simulink model "bustestsysa"  (Simulink 9.3)
settings: Solver=ode15s  StartTime=0.0  StopTime=0.08  RelTol=1e-3  AbsTol=1e-6
libraries: powerlib x113
settings Model: Creator=Dr. Lotfifard  LastModifiedBy=renji  ExtModeTrigMode=oneshot  ExtModeArmWhenConnect=off
settings SolverCC: AutoScaleAbsTol=off
settings OptimizationCC: BlockReduction=off  BooleanDataType=off  ExpressionDepthLimit=2147483647
settings DebuggingCC: SaveWithParameterizedLinksMsg=none  SignalResolutionControl=TryResolveAllWithWarning  MultiTaskDSMMsg=warning  MultiTaskCondExecSysMsg=none  StateNameClashWarn=warning
settings HardwareCC: TargetUnknown=on
settings GRTTargetCC: GeneratePreprocessorConditionals=Disable all
settings SimscapeCC: SimscapeNormalizeSystem=off

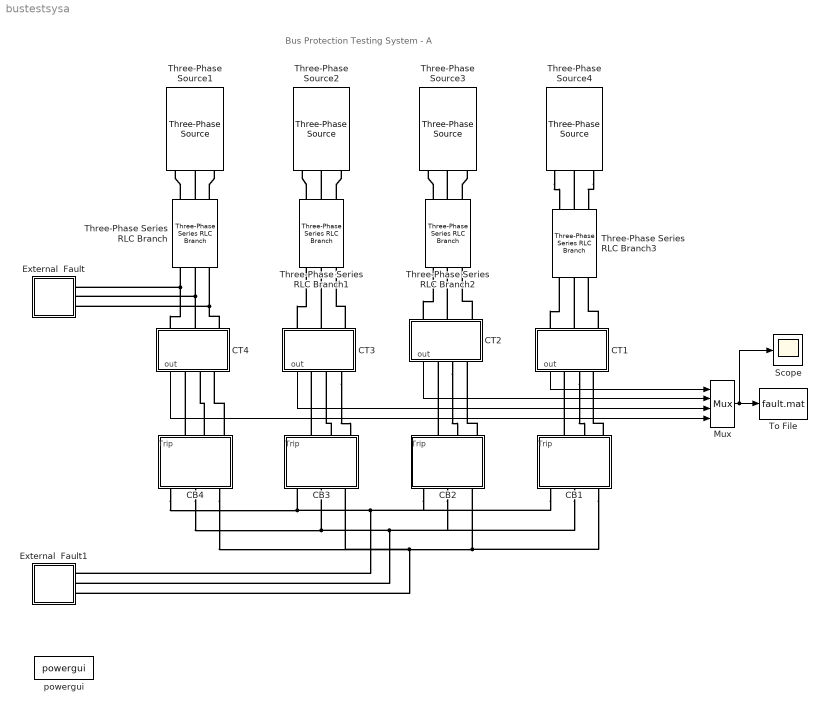
== system bustestsysa ==
  note: Bus Protection Testing System - A
  CB1 : Subsystem
  CB2 : Subsystem
  CB3 : Subsystem
  CB4 : Subsystem
  CT1 : Subsystem  mask(3-phase Current Transformer){pf=[6000 60 ], urx1=[5  0.002 0.08 ], urx2=[2000 0.002 0.08], sat=[0 0; 1 1.1; 2 1.2; 1000 1.3; 10000 1.35; 100000 1.4], Rm=1, phi0='auto'}
      mask prompts: pf "[Three-phase rated power(VA)  Frequency (Hz)]"; urx1 "Winding 1 (Yg) :    [Ph-Ph Voltage(Vrms)  R(pu)  X(pu)] :"; urx2 "Winding 2 (Yg) :    [Ph-Ph voltage(Vrms)  R(pu)  X(pu)] :"; sat "Saturation characterstic [i1(pu) phi1(pu); i2 phi2; ...]"; Rm "Core loss resistance Rm (pu) :"; phi0 "Residual fluxes (pu)  [phi0A  phi0B phi0C] or 'auto'"
      mask help:
      | This block implements a three phase Saturable transformer by using three mono-phase saturable transformers.
      | Winding one is connected in Y configuration with neutral connected to the ground.
      | Winding two is connected in Y configuration with neutral connected to ground.
      | Enter the saturation characteristic for one mono-phase saturable transformer. The saturation characteristic is the same for A,B, and C  phases.
      | For flux initialization, you  can either specify a vector of three resisual fluxes, or use automatic initialization  corresponding to steady state by entering the string 'auto'.
      mask init:
      | pnom=pf(1)/3; fnom=pf(2);
      | u1=urx1(1)/sqrt(3); r1=urx1(2); x1=urx1(3);
      | u2=urx2(1)/sqrt(3); r2=urx2(2); x2=urx2(3);
      | if  isstr(phi0) & strcmp(phi0,'auto')
      |    Rm_phi0_1=Rm;
      |    Rm_phi0_2=Rm;
      |    Rm_phi0_3=Rm;
      | else
      |    Rm_phi0_1=[Rm phi0(1)];
      |    Rm_phi0_2=[Rm phi0(2)];
      |    Rm_phi0_3=[Rm phi0(3)];
      | end
  CT2 : Subsystem  mask(3-phase Current Transformer){pf=[6000 60 ], urx1=[5  0.002 0.08 ], urx2=[2000 0.002 0.08], sat=[0 0; 1 1.1; 2 1.2; 1000 1.3; 10000 1.35; 100000 1.4], Rm=1, phi0='auto'}
      mask prompts: pf "[Three-phase rated power(VA)  Frequency (Hz)]"; urx1 "Winding 1 (Yg) :    [Ph-Ph Voltage(Vrms)  R(pu)  X(pu)] :"; urx2 "Winding 2 (Yg) :    [Ph-Ph voltage(Vrms)  R(pu)  X(pu)] :"; sat "Saturation characterstic [i1(pu) phi1(pu); i2 phi2; ...]"; Rm "Core loss resistance Rm (pu) :"; phi0 "Residual fluxes (pu)  [phi0A  phi0B phi0C] or 'auto'"
      mask help:
      | This block implements a three phase Saturable transformer by using three mono-phase saturable transformers.
      | Winding one is connected in Y configuration with neutral connected to the ground.
      | Winding two is connected in Y configuration with neutral connected to ground.
      | Enter the saturation characteristic for one mono-phase saturable transformer. The saturation characteristic is the same for A,B, and C  phases.
      | For flux initialization, you  can either specify a vector of three resisual fluxes, or use automatic initialization  corresponding to steady state by entering the string 'auto'.
      mask init: same as bustestsysa/CT1
  CT3 : Subsystem  mask(3-phase Current Transformer){pf=[6000 60 ], urx1=[5  0.002 0.08 ], urx2=[2000 0.002 0.08], sat=[0 0; 1 1.1; 2 1.2; 1000 1.3; 10000 1.35; 100000 1.4], Rm=1, phi0='auto'}
      mask prompts: pf "[Three-phase rated power(VA)  Frequency (Hz)]"; urx1 "Winding 1 (Yg) :    [Ph-Ph Voltage(Vrms)  R(pu)  X(pu)] :"; urx2 "Winding 2 (Yg) :    [Ph-Ph voltage(Vrms)  R(pu)  X(pu)] :"; sat "Saturation characterstic [i1(pu) phi1(pu); i2 phi2; ...]"; Rm "Core loss resistance Rm (pu) :"; phi0 "Residual fluxes (pu)  [phi0A  phi0B phi0C] or 'auto'"
      mask help:
      | This block implements a three phase Saturable transformer by using three mono-phase saturable transformers.
      | Winding one is connected in Y configuration with neutral connected to the ground.
      | Winding two is connected in Y configuration with neutral connected to ground.
      | Enter the saturation characteristic for one mono-phase saturable transformer. The saturation characteristic is the same for A,B, and C  phases.
      | For flux initialization, you  can either specify a vector of three resisual fluxes, or use automatic initialization  corresponding to steady state by entering the string 'auto'.
      mask init: same as bustestsysa/CT1
  CT4 : Subsystem  mask(3-phase Current Transformer){pf=[6000 60 ], urx1=[5  0.002 0.08 ], urx2=[2000 0.002 0.08], sat=[0 0; 1 1.1; 2 1.2; 1000 1.3; 10000 1.35; 100000 1.4], Rm=1, phi0='auto'}
      mask prompts: pf "[Three-phase rated power(VA)  Frequency (Hz)]"; urx1 "Winding 1 (Yg) :    [Ph-Ph Voltage(Vrms)  R(pu)  X(pu)] :"; urx2 "Winding 2 (Yg) :    [Ph-Ph voltage(Vrms)  R(pu)  X(pu)] :"; sat "Saturation characterstic [i1(pu) phi1(pu); i2 phi2; ...]"; Rm "Core loss resistance Rm (pu) :"; phi0 "Residual fluxes (pu)  [phi0A  phi0B phi0C] or 'auto'"
      mask help:
      | This block implements a three phase Saturable transformer by using three mono-phase saturable transformers.
      | Winding one is connected in Y configuration with neutral connected to the ground.
      | Winding two is connected in Y configuration with neutral connected to ground.
      | Enter the saturation characteristic for one mono-phase saturable transformer. The saturation characteristic is the same for A,B, and C  phases.
      | For flux initialization, you  can either specify a vector of three resisual fluxes, or use automatic initialization  corresponding to steady state by entering the string 'auto'.
      mask init: same as bustestsysa/CT1
  External  Fault : Subsystem  mask{Tfault=0.2}
      mask prompts: Tfault "Fault time (in sec.)"
      mask Display: plot(0,0,100,100,[44,47,56,38,50],[23,8,64,44,97],[56,47],[25,8])
  External  Fault1 : Subsystem  mask{Tfault=0.02}
      mask prompts: Tfault "Fault time (in sec.)"
      mask Display: plot(0,0,100,100,[44,47,56,38,50],[23,8,64,44,97],[56,47],[25,8])
  Mux : Mux
  Scope : Scope
  Three-Phase Series RLC Branch : powerlib/Elements/Three-Phase Series RLC Branch  LConnTagsString=A|B|C  RConnTagsString=A|B|C  BranchType=RL  Resistance=2  Inductance=0.1  Capacitance=1e-6  Measurements=None
      settings: SourceProductName=Simscape Electrical
  Three-Phase Series RLC Branch1 : powerlib/Elements/Three-Phase Series RLC Branch  LConnTagsString=A|B|C  RConnTagsString=A|B|C  BranchType=RL  Resistance=2  Inductance=0.12  Capacitance=1e-6  Measurements=None
      settings: SourceProductName=Simscape Electrical
  Three-Phase Series RLC Branch2 : powerlib/Elements/Three-Phase Series RLC Branch  LConnTagsString=A|B|C  RConnTagsString=A|B|C  BranchType=RL  Resistance=4  Inductance=0.5  Capacitance=1e-6  Measurements=None
      settings: SourceProductName=Simscape Electrical
  Three-Phase Series RLC Branch3 : powerlib/Elements/Three-Phase Series RLC Branch  LConnTagsString=A|B|C  RConnTagsString=A|B|C  BranchType=RL  Resistance=4  Inductance=0.6  Capacitance=1e-6  Measurements=None
      settings: SourceProductName=Simscape Electrical
  Three-Phase Source1 : powerlib/Electrical Sources/Three-Phase Source  InternalConnection=Yg  VoltagePhases=off  Voltage=510e3/sqrt(3)*sqrt(2)  PhaseAngle=0  Voltage_phases=[25e3 25e3 25e3]/sqrt(3)  PhaseAngles_phases=[0 -120 +120]  Frequency=60  NonIdealSource=on  SpecifyImpedance=off  Resistance=0.1  Inductance=20e-3  ShortCircuitLevel=100e6  BaseVoltage=25e3  XRratio=7  BusType=swing  Pref=0  Qref=0  Prefabc=[10e3, 10e3, 10e3]  Qrefabc=[0, 0, 0]  Qmin=-inf  Qmax=inf
      settings: SourceProductName=Simscape Electrical
  Three-Phase Source2 : powerlib/Electrical Sources/Three-Phase Source  InternalConnection=Yg  VoltagePhases=off  Voltage=500e3/sqrt(3)*sqrt(2)  PhaseAngle=-10  Voltage_phases=[25e3 25e3 25e3]/sqrt(3)  PhaseAngles_phases=[0 -120 +120]  Frequency=60  NonIdealSource=on  SpecifyImpedance=off  Resistance=0.1  Inductance=20e-3  ShortCircuitLevel=100e6  BaseVoltage=25e3  XRratio=7  BusType=swing  Pref=0  Qref=0  Prefabc=[10e3, 10e3, 10e3]  Qrefabc=[0, 0, 0]  Qmin=-inf  Qmax=inf
      settings: SourceProductName=Simscape Electrical
  Three-Phase Source3 : powerlib/Electrical Sources/Three-Phase Source  InternalConnection=Yg  VoltagePhases=off  Voltage=520e3/sqrt(3)*sqrt(2)  PhaseAngle=20  Voltage_phases=[25e3 25e3 25e3]/sqrt(3)  PhaseAngles_phases=[0 -120 +120]  Frequency=60  NonIdealSource=on  SpecifyImpedance=off  Resistance=0.1  Inductance=20e-3  ShortCircuitLevel=100e6  BaseVoltage=25e3  XRratio=7  BusType=swing  Pref=0  Qref=0  Prefabc=[10e3, 10e3, 10e3]  Qrefabc=[0, 0, 0]  Qmin=-inf  Qmax=inf
      settings: SourceProductName=Simscape Electrical
  Three-Phase Source4 : powerlib/Electrical Sources/Three-Phase Source  InternalConnection=Yg  VoltagePhases=off  Voltage=520e3/sqrt(3)*sqrt(2)  PhaseAngle=20  Voltage_phases=[25e3 25e3 25e3]/sqrt(3)  PhaseAngles_phases=[0 -120 +120]  Frequency=60  NonIdealSource=on  SpecifyImpedance=off  Resistance=0.1  Inductance=20e-3  ShortCircuitLevel=100e6  BaseVoltage=25e3  XRratio=7  BusType=swing  Pref=0  Qref=0  Prefabc=[10e3, 10e3, 10e3]  Qrefabc=[0, 0, 0]  Qmin=-inf  Qmax=inf
      settings: SourceProductName=Simscape Electrical
  To File : ToFile  Filename=fault.mat  MatrixName=i
  powergui : powerlib/powergui  SimulationMode=Continuous  SampleTime=0  frequency=60  Iterations=50  frequencyindice=0  Pbase=100e6  ErrMax=1e-4  UnitsV=kV  UnitsW=MW  buscounter=0  FunctionMessages=off  echomessages=off  EnableUseOfTLC=off  CurrentSourceSwitches=on  DisableSnubberDevices=off  DisableRonSwitches=off  DisableVfSwitches=off  DisplayEquations=off  AutomaticDiscreteSolvers=off  SolverType=Tustin/Backward Euler (TBE)  Interpol=off  ExternalGateDelay=off  methode=off  Ts=0  x0status=blocks  SPID=off  SwTol=0  HookPort=off  NonlinearTolerance=0  nMaxIteration=15  ContinueOnMaxIteration=off  RestoreLinks=warning  ResistiveCurrentMeasurement=off  Frange=[0:2:500]  Ylog=off  Xlog=on  ShowGrid=off  save=off  variable=ZData  structure=0  ZoomFFT=on  StartTime=0.0  cycles=1  DisplayStyle=1  fundamental=60  FreqAxis=off  MaxFrequency=1000  frequencyindicesteady=1  RmsSteady=1  display=off
      settings: SourceProductName=Simscape Electrical
  wires:
  Mux/1 -> To File/1, Scope/1
  CT1/1(out) -> Mux/1
  CT4/1(out) -> Mux/4
  CT3/1(out) -> Mux/3
  CT2/1(out) -> Mux/2
  connections:
  Three-Phase Series RLC Branch1/RConn3 -- Three-Phase Source2/RConn3
  CB4/LConn1 -- CT4/RConn1
  CB4/LConn2 -- CT4/RConn2
  CB4/LConn3 -- CT4/RConn3
  CB3/LConn1 -- CT3/RConn1
  CB3/LConn2 -- CT3/RConn2
  CT3/RConn3 -- CB3/LConn3
  CB2/LConn1 -- CT2/RConn1
  CT2/RConn2 -- CB2/LConn2
  CB2/LConn3 -- CT2/RConn3
  CB1/LConn1 -- CT1/RConn1
  CT1/RConn2 -- CB1/LConn2
  CB1/LConn3 -- CT1/RConn3
  CB2/RConn1 -- CB1/RConn1 -- CB4/RConn1 -- CB3/RConn1 -- External  Fault1/LConn1
  CB2/RConn2 -- CB1/RConn2 -- CB4/RConn2 -- CB3/RConn2 -- External  Fault1/LConn2
  CB4/RConn3 -- CB3/RConn3 -- CB2/RConn3 -- CB1/RConn3 -- External  Fault1/LConn3
  CT1/LConn1 -- Three-Phase Series RLC Branch3/LConn1
  CT1/LConn2 -- Three-Phase Series RLC Branch3/LConn2
  CT1/LConn3 -- Three-Phase Series RLC Branch3/LConn3
  CT2/LConn3 -- Three-Phase Series RLC Branch2/LConn3
  CT2/LConn2 -- Three-Phase Series RLC Branch2/LConn2
  CT2/LConn1 -- Three-Phase Series RLC Branch2/LConn1
  CT3/LConn3 -- Three-Phase Series RLC Branch1/LConn3
  CT3/LConn2 -- Three-Phase Series RLC Branch1/LConn2
  CT3/LConn1 -- Three-Phase Series RLC Branch1/LConn1
  CT4/LConn3 -- Three-Phase Series RLC Branch/LConn3 -- External  Fault/LConn3
  CT4/LConn2 -- Three-Phase Series RLC Branch/LConn2 -- External  Fault/LConn2
  CT4/LConn1 -- Three-Phase Series RLC Branch/LConn1 -- External  Fault/LConn1
  Three-Phase Series RLC Branch/RConn3 -- Three-Phase Source1/RConn3
  Three-Phase Series RLC Branch/RConn2 -- Three-Phase Source1/RConn2
  Three-Phase Series RLC Branch/RConn1 -- Three-Phase Source1/RConn1
  Three-Phase Series RLC Branch3/RConn2 -- Three-Phase Source4/RConn2
  Three-Phase Source4/RConn1 -- Three-Phase Series RLC Branch3/RConn1
  Three-Phase Source4/RConn3 -- Three-Phase Series RLC Branch3/RConn3
  Three-Phase Series RLC Branch2/RConn3 -- Three-Phase Source3/RConn3
  Three-Phase Series RLC Branch2/RConn2 -- Three-Phase Source3/RConn2
  Three-Phase Series RLC Branch2/RConn1 -- Three-Phase Source3/RConn1
  Three-Phase Series RLC Branch1/RConn2 -- Three-Phase Source2/RConn2
  Three-Phase Series RLC Branch1/RConn1 -- Three-Phase Source2/RConn1

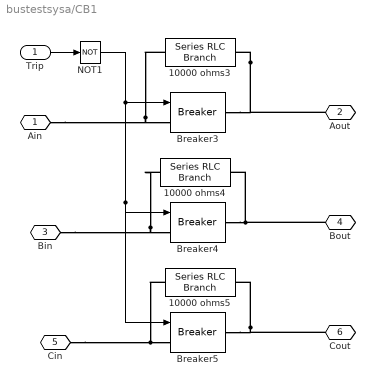
== system bustestsysa/CB1 ==
  Trip : Inport
  10000 ohms3 : powerlib/Elements/Series RLC Branch  LConnTagsString=__new0  RConnTagsString=__new0  BranchType=R  Resistance=10000  Inductance=1e-3  SetiL0=off  InitialCurrent=0  Capacitance=1e-6  Setx0=off  InitialVoltage=0  Measurements=None
      settings: SourceProductName=Simscape Electrical
  10000 ohms4 : powerlib/Elements/Series RLC Branch  LConnTagsString=__new0  RConnTagsString=__new0  BranchType=R  Resistance=10000  Inductance=1e-3  SetiL0=off  InitialCurrent=0  Capacitance=1e-6  Setx0=off  InitialVoltage=0  Measurements=None
      settings: SourceProductName=Simscape Electrical
  10000 ohms5 : powerlib/Elements/Series RLC Branch  LConnTagsString=__new0  RConnTagsString=__new0  BranchType=R  Resistance=10000  Inductance=1e-3  SetiL0=off  InitialCurrent=0  Capacitance=1e-6  Setx0=off  InitialVoltage=0  Measurements=None
      settings: SourceProductName=Simscape Electrical
  Breaker3 : powerlib/Elements/Breaker  InitialState=1  SwitchingTimes="[ 1/60  5/60 ]"  External=on  BreakerResistance=0.01  SnubberResistance=1e6  SnubberCapacitance=inf  Measurements=None  MoreParameters=off  NoBreakLoop=off
      settings: SourceProductName=Simscape Electrical
  Breaker4 : powerlib/Elements/Breaker  InitialState=1  SwitchingTimes="[ 1/60  5/60 ]"  External=on  BreakerResistance=0.01  SnubberResistance=1e6  SnubberCapacitance=inf  Measurements=None  MoreParameters=off  NoBreakLoop=off
      settings: SourceProductName=Simscape Electrical
  Breaker5 : powerlib/Elements/Breaker  InitialState=1  SwitchingTimes="[ 1/60  5/60 ]"  External=on  BreakerResistance=0.01  SnubberResistance=1e6  SnubberCapacitance=inf  Measurements=None  MoreParameters=off  NoBreakLoop=off
      settings: SourceProductName=Simscape Electrical
  NOT1 : Logic  Operator=NOT  Inputs=1
  Ain : PMIOPort  Side=Left
  Aout : PMIOPort  Port=2  Side=Right
  Bin : PMIOPort  Port=3  Side=Left
  Bout : PMIOPort  Port=4  Side=Right
  Cin : PMIOPort  Port=5  Side=Left
  Cout : PMIOPort  Port=6  Side=Right
  wires:
  Trip/1 -> NOT1/1
  NOT1/1 -> Breaker3/1, Breaker4/1, Breaker5/1
  connections:
  Ain/RConn1 -- Breaker3/LConn1 -- 10000 ohms3/LConn1
  Aout/RConn1 -- Breaker3/RConn1 -- 10000 ohms3/RConn1
  Bin/RConn1 -- Breaker4/LConn1 -- 10000 ohms4/LConn1
  Bout/RConn1 -- Breaker4/RConn1 -- 10000 ohms4/RConn1
  Cin/RConn1 -- Breaker5/LConn1 -- 10000 ohms5/LConn1
  Cout/RConn1 -- Breaker5/RConn1 -- 10000 ohms5/RConn1

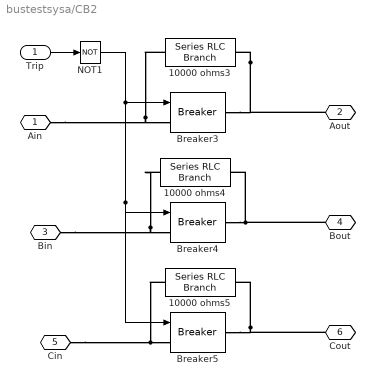
== system bustestsysa/CB2 ==
  Trip : Inport
  10000 ohms3 : powerlib/Elements/Series RLC Branch  LConnTagsString=__new0  RConnTagsString=__new0  BranchType=R  Resistance=10000  Inductance=1e-3  SetiL0=off  InitialCurrent=0  Capacitance=1e-6  Setx0=off  InitialVoltage=0  Measurements=None
      settings: SourceProductName=Simscape Electrical
  10000 ohms4 : powerlib/Elements/Series RLC Branch  LConnTagsString=__new0  RConnTagsString=__new0  BranchType=R  Resistance=10000  Inductance=1e-3  SetiL0=off  InitialCurrent=0  Capacitance=1e-6  Setx0=off  InitialVoltage=0  Measurements=None
      settings: SourceProductName=Simscape Electrical
  10000 ohms5 : powerlib/Elements/Series RLC Branch  LConnTagsString=__new0  RConnTagsString=__new0  BranchType=R  Resistance=10000  Inductance=1e-3  SetiL0=off  InitialCurrent=0  Capacitance=1e-6  Setx0=off  InitialVoltage=0  Measurements=None
      settings: SourceProductName=Simscape Electrical
  Breaker3 : powerlib/Elements/Breaker  InitialState=0  SwitchingTimes="[ 1/60  5/60 ]"  External=on  BreakerResistance=0.01  SnubberResistance=1e6  SnubberCapacitance=inf  Measurements=None  MoreParameters=off  NoBreakLoop=off
      settings: SourceProductName=Simscape Electrical
  Breaker4 : powerlib/Elements/Breaker  InitialState=0  SwitchingTimes="[ 1/60  5/60 ]"  External=on  BreakerResistance=0.01  SnubberResistance=1e6  SnubberCapacitance=inf  Measurements=None  MoreParameters=off  NoBreakLoop=off
      settings: SourceProductName=Simscape Electrical
  Breaker5 : powerlib/Elements/Breaker  InitialState=0  SwitchingTimes="[ 1/60  5/60 ]"  External=on  BreakerResistance=0.01  SnubberResistance=1e6  SnubberCapacitance=inf  Measurements=None  MoreParameters=off  NoBreakLoop=off
      settings: SourceProductName=Simscape Electrical
  NOT1 : Logic  Operator=NOT  Inputs=1
  Ain : PMIOPort  Side=Left
  Aout : PMIOPort  Port=2  Side=Right
  Bin : PMIOPort  Port=3  Side=Left
  Bout : PMIOPort  Port=4  Side=Right
  Cin : PMIOPort  Port=5  Side=Left
  Cout : PMIOPort  Port=6  Side=Right
  wires:
  Trip/1 -> NOT1/1
  NOT1/1 -> Breaker3/1, Breaker4/1, Breaker5/1
  connections:
  Ain/RConn1 -- Breaker3/LConn1 -- 10000 ohms3/LConn1
  Aout/RConn1 -- Breaker3/RConn1 -- 10000 ohms3/RConn1
  Bin/RConn1 -- Breaker4/LConn1 -- 10000 ohms4/LConn1
  Bout/RConn1 -- Breaker4/RConn1 -- 10000 ohms4/RConn1
  Cin/RConn1 -- Breaker5/LConn1 -- 10000 ohms5/LConn1
  Cout/RConn1 -- Breaker5/RConn1 -- 10000 ohms5/RConn1

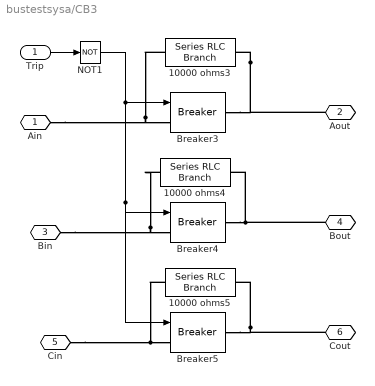
== system bustestsysa/CB3 ==
  Trip : Inport
  10000 ohms3 : powerlib/Elements/Series RLC Branch  LConnTagsString=__new0  RConnTagsString=__new0  BranchType=R  Resistance=10000  Inductance=1e-3  SetiL0=off  InitialCurrent=0  Capacitance=1e-6  Setx0=off  InitialVoltage=0  Measurements=None
      settings: SourceProductName=Simscape Electrical
  10000 ohms4 : powerlib/Elements/Series RLC Branch  LConnTagsString=__new0  RConnTagsString=__new0  BranchType=R  Resistance=10000  Inductance=1e-3  SetiL0=off  InitialCurrent=0  Capacitance=1e-6  Setx0=off  InitialVoltage=0  Measurements=None
      settings: SourceProductName=Simscape Electrical
  10000 ohms5 : powerlib/Elements/Series RLC Branch  LConnTagsString=__new0  RConnTagsString=__new0  BranchType=R  Resistance=10000  Inductance=1e-3  SetiL0=off  InitialCurrent=0  Capacitance=1e-6  Setx0=off  InitialVoltage=0  Measurements=None
      settings: SourceProductName=Simscape Electrical
  Breaker3 : powerlib/Elements/Breaker  InitialState=1  SwitchingTimes="[ 1/60  5/60 ]"  External=on  BreakerResistance=0.01  SnubberResistance=1e6  SnubberCapacitance=inf  Measurements=None  MoreParameters=off  NoBreakLoop=off
      settings: SourceProductName=Simscape Electrical
  Breaker4 : powerlib/Elements/Breaker  InitialState=1  SwitchingTimes="[ 1/60  5/60 ]"  External=on  BreakerResistance=0.01  SnubberResistance=1e6  SnubberCapacitance=inf  Measurements=None  MoreParameters=off  NoBreakLoop=off
      settings: SourceProductName=Simscape Electrical
  Breaker5 : powerlib/Elements/Breaker  InitialState=1  SwitchingTimes="[ 1/60  5/60 ]"  External=on  BreakerResistance=0.01  SnubberResistance=1e6  SnubberCapacitance=inf  Measurements=None  MoreParameters=off  NoBreakLoop=off
      settings: SourceProductName=Simscape Electrical
  NOT1 : Logic  Operator=NOT  Inputs=1
  Ain : PMIOPort  Side=Left
  Aout : PMIOPort  Port=2  Side=Right
  Bin : PMIOPort  Port=3  Side=Left
  Bout : PMIOPort  Port=4  Side=Right
  Cin : PMIOPort  Port=5  Side=Left
  Cout : PMIOPort  Port=6  Side=Right
  wires:
  Trip/1 -> NOT1/1
  NOT1/1 -> Breaker3/1, Breaker4/1, Breaker5/1
  connections:
  Ain/RConn1 -- Breaker3/LConn1 -- 10000 ohms3/LConn1
  Aout/RConn1 -- Breaker3/RConn1 -- 10000 ohms3/RConn1
  Bin/RConn1 -- Breaker4/LConn1 -- 10000 ohms4/LConn1
  Bout/RConn1 -- Breaker4/RConn1 -- 10000 ohms4/RConn1
  Cin/RConn1 -- Breaker5/LConn1 -- 10000 ohms5/LConn1
  Cout/RConn1 -- Breaker5/RConn1 -- 10000 ohms5/RConn1

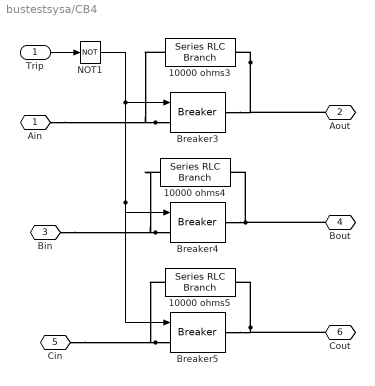
== system bustestsysa/CB4 ==
  Trip : Inport
  10000 ohms3 : powerlib/Elements/Series RLC Branch  LConnTagsString=__new0  RConnTagsString=__new0  BranchType=R  Resistance=10000  Inductance=1e-3  SetiL0=off  InitialCurrent=0  Capacitance=1e-6  Setx0=off  InitialVoltage=0  Measurements=None
      settings: SourceProductName=Simscape Electrical
  10000 ohms4 : powerlib/Elements/Series RLC Branch  LConnTagsString=__new0  RConnTagsString=__new0  BranchType=R  Resistance=10000  Inductance=1e-3  SetiL0=off  InitialCurrent=0  Capacitance=1e-6  Setx0=off  InitialVoltage=0  Measurements=None
      settings: SourceProductName=Simscape Electrical
  10000 ohms5 : powerlib/Elements/Series RLC Branch  LConnTagsString=__new0  RConnTagsString=__new0  BranchType=R  Resistance=10000  Inductance=1e-3  SetiL0=off  InitialCurrent=0  Capacitance=1e-6  Setx0=off  InitialVoltage=0  Measurements=None
      settings: SourceProductName=Simscape Electrical
  Breaker3 : powerlib/Elements/Breaker  InitialState=1  SwitchingTimes="[ 1/60  5/60 ]"  External=on  BreakerResistance=0.01  SnubberResistance=1e6  SnubberCapacitance=inf  Measurements=None  MoreParameters=off  NoBreakLoop=off
      settings: SourceProductName=Simscape Electrical
  Breaker4 : powerlib/Elements/Breaker  InitialState=1  SwitchingTimes="[ 1/60  5/60 ]"  External=on  BreakerResistance=0.01  SnubberResistance=1e6  SnubberCapacitance=inf  Measurements=None  MoreParameters=off  NoBreakLoop=off
      settings: SourceProductName=Simscape Electrical
  Breaker5 : powerlib/Elements/Breaker  InitialState=1  SwitchingTimes="[ 1/60  5/60 ]"  External=on  BreakerResistance=0.01  SnubberResistance=1e6  SnubberCapacitance=inf  Measurements=None  MoreParameters=off  NoBreakLoop=off
      settings: SourceProductName=Simscape Electrical
  NOT1 : Logic  Operator=NOT  Inputs=1
  Ain : PMIOPort  Side=Left
  Aout : PMIOPort  Port=2  Side=Right
  Bin : PMIOPort  Port=3  Side=Left
  Bout : PMIOPort  Port=4  Side=Right
  Cin : PMIOPort  Port=5  Side=Left
  Cout : PMIOPort  Port=6  Side=Right
  wires:
  Trip/1 -> NOT1/1
  NOT1/1 -> Breaker3/1, Breaker4/1, Breaker5/1
  connections:
  Breaker3/LConn1 -- 10000 ohms3/LConn1 -- Ain/RConn1
  Breaker3/RConn1 -- 10000 ohms3/RConn1 -- Aout/RConn1
  Breaker4/LConn1 -- 10000 ohms4/LConn1 -- Bin/RConn1
  Breaker4/RConn1 -- 10000 ohms4/RConn1 -- Bout/RConn1
  Breaker5/LConn1 -- 10000 ohms5/LConn1 -- Cin/RConn1
  Breaker5/RConn1 -- 10000 ohms5/RConn1 -- Cout/RConn1

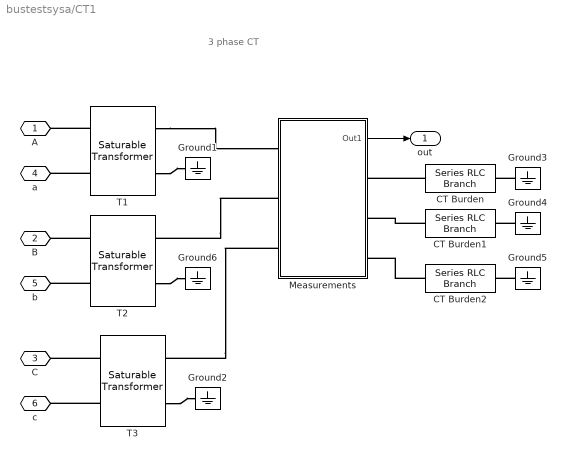
== system bustestsysa/CT1 ==
  note: 3 phase CT
  CT Burden : powerlib/Elements/Series RLC Branch  LConnTagsString=__new0  RConnTagsString=__new0  BranchType=RL  Resistance=3  Inductance=1e-3  SetiL0=off  InitialCurrent=0  Capacitance=1e-6  Setx0=off  InitialVoltage=0  Measurements=None
      settings: SourceProductName=Simscape Electrical
  CT Burden1 : powerlib/Elements/Series RLC Branch  LConnTagsString=__new0  RConnTagsString=__new0  BranchType=RL  Resistance=3  Inductance=1e-3  SetiL0=off  InitialCurrent=0  Capacitance=1e-6  Setx0=off  InitialVoltage=0  Measurements=None
      settings: SourceProductName=Simscape Electrical
  CT Burden2 : powerlib/Elements/Series RLC Branch  LConnTagsString=__new0  RConnTagsString=__new0  BranchType=RL  Resistance=3  Inductance=1e-3  SetiL0=off  InitialCurrent=0  Capacitance=1e-6  Setx0=off  InitialVoltage=0  Measurements=None
      settings: SourceProductName=Simscape Electrical
  Ground{1..6} (6 alike) : powerlib/Elements/Ground  LConnTagsString=a
      settings: SourceProductName=Simscape Electrical
  Measurements : Subsystem  mask(3 Phase Current Measurement){}
  T1 : powerlib/Elements/Saturable Transformer  ThreeWindings=off  Hysteresis=off  DataFile='hysteresis.mat'  Measurements=None  UNITS=pu  NominalPower=[pnom fnom]  Winding1=[u1 r1 x1]  Winding2=[u2 r2 x2]  Winding3=[u2 r2 x2]  Saturation=sat  CoreLoss=Rm_phi0_1  BreakLoop=off  DiscreteSolver=Trapezoidal iterative  DataType=off  InitialFlux=-4.24024745954317e-05  TransfoNumber=1
      settings: SourceProductName=Simscape Electrical  SourceProductBaseCode=PS
  T2 : powerlib/Elements/Saturable Transformer  ThreeWindings=off  Hysteresis=off  DataFile='hysteresis.mat'  Measurements=None  UNITS=pu  NominalPower=[pnom fnom]  Winding1=[u1 r1 x1]  Winding2=[u2 r2 x2]  Winding3=[u2 r2 x2]  Saturation=sat  CoreLoss=Rm_phi0_1  BreakLoop=off  DiscreteSolver=Trapezoidal iterative  DataType=off  InitialFlux=-0.00041396463872332  TransfoNumber=1
      settings: SourceProductName=Simscape Electrical  SourceProductBaseCode=PS
  T3 : powerlib/Elements/Saturable Transformer  ThreeWindings=off  Hysteresis=off  DataFile='hysteresis.mat'  Measurements=None  UNITS=pu  NominalPower=[pnom fnom]  Winding1=[u1 r1 x1]  Winding2=[u2 r2 x2]  Winding3=[u2 r2 x2]  Saturation=sat  CoreLoss=Rm_phi0_1  BreakLoop=off  DiscreteSolver=Trapezoidal iterative  DataType=off  InitialFlux=0.000456367113318769  TransfoNumber=1
      settings: SourceProductName=Simscape Electrical  SourceProductBaseCode=PS
  A : PMIOPort  Side=Left
  B : PMIOPort  Port=2  Side=Left
  C : PMIOPort  Port=3  Side=Left
  a : PMIOPort  Port=4  Side=Right
  b : PMIOPort  Port=5  Side=Right
  c : PMIOPort  Port=6  Side=Right
  out : Outport  InitialOutput=0
  wires:
  Measurements/1(Out1) -> out/1
  connections:
  Ground3/LConn1 -- CT Burden/RConn1
  Ground4/LConn1 -- CT Burden1/RConn1
  Ground5/LConn1 -- CT Burden2/RConn1
  T1/RConn2 -- Ground1/LConn1
  T2/RConn2 -- Ground6/LConn1
  T3/RConn2 -- Ground2/LConn1
  CT Burden/LConn1 -- Measurements/RConn1
  CT Burden1/LConn1 -- Measurements/RConn2
  CT Burden2/LConn1 -- Measurements/RConn3
  T1/RConn1 -- Measurements/LConn1
  Measurements/LConn2 -- T2/RConn1
  Measurements/LConn3 -- T3/RConn1
  T1/LConn1 -- A/RConn1
  T2/LConn1 -- B/RConn1
  T3/LConn1 -- C/RConn1
  T3/LConn2 -- c/RConn1
  T2/LConn2 -- b/RConn1
  T1/LConn2 -- a/RConn1

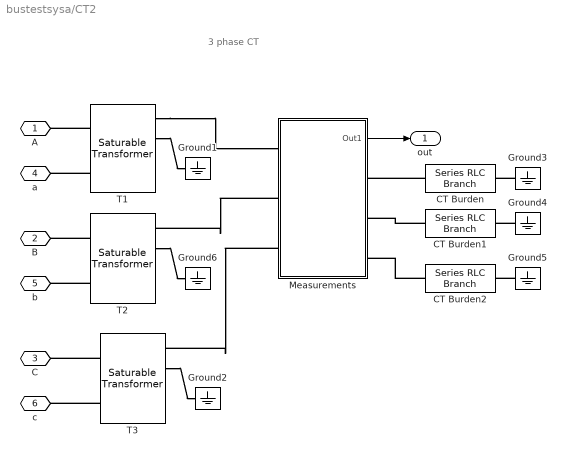
== system bustestsysa/CT2 ==
  note: 3 phase CT
  CT Burden : powerlib/Elements/Series RLC Branch  LConnTagsString=__new0  RConnTagsString=__new0  BranchType=RL  Resistance=3  Inductance=1e-3  SetiL0=off  InitialCurrent=0  Capacitance=1e-6  Setx0=off  InitialVoltage=0  Measurements=None
      settings: SourceProductName=Simscape Electrical
  CT Burden1 : powerlib/Elements/Series RLC Branch  LConnTagsString=__new0  RConnTagsString=__new0  BranchType=RL  Resistance=3  Inductance=1e-3  SetiL0=off  InitialCurrent=0  Capacitance=1e-6  Setx0=off  InitialVoltage=0  Measurements=None
      settings: SourceProductName=Simscape Electrical
  CT Burden2 : powerlib/Elements/Series RLC Branch  LConnTagsString=__new0  RConnTagsString=__new0  BranchType=RL  Resistance=3  Inductance=1e-3  SetiL0=off  InitialCurrent=0  Capacitance=1e-6  Setx0=off  InitialVoltage=0  Measurements=None
      settings: SourceProductName=Simscape Electrical
  Ground{1..6} (6 alike) : powerlib/Elements/Ground  LConnTagsString=a
      settings: SourceProductName=Simscape Electrical
  Measurements : Subsystem  mask(3 Phase Current Measurement){}
  T1 : powerlib/Elements/Saturable Transformer  ThreeWindings=off  Hysteresis=off  DataFile='hysteresis.mat'  Measurements=None  UNITS=pu  NominalPower=[pnom fnom]  Winding1=[u1 r1 x1]  Winding2=[u2 r2 x2]  Winding3=0  Saturation=sat  CoreLoss=Rm_phi0_1  BreakLoop=off  DiscreteSolver=Trapezoidal iterative  DataType=off  InitialFlux=1.18112582847913e-05  TransfoNumber=1
      settings: SourceProductName=Simscape Electrical  SourceProductBaseCode=PS
  T2 : powerlib/Elements/Saturable Transformer  ThreeWindings=off  Hysteresis=off  DataFile='hysteresis.mat'  Measurements=None  UNITS=pu  NominalPower=[pnom fnom]  Winding1=[u1 r1 x1]  Winding2=[u2 r2 x2]  Winding3=[u2 r2 x2]  Saturation=sat  CoreLoss=Rm_phi0_1  BreakLoop=off  DiscreteSolver=Trapezoidal iterative  DataType=off  InitialFlux=-7.15518015200205e-06  TransfoNumber=1
      settings: SourceProductName=Simscape Electrical  SourceProductBaseCode=PS
  T3 : powerlib/Elements/Saturable Transformer  ThreeWindings=off  Hysteresis=off  DataFile='hysteresis.mat'  Measurements=None  UNITS=pu  NominalPower=[pnom fnom]  Winding1=[u1 r1 x1]  Winding2=[u2 r2 x2]  Winding3=[u2 r2 x2]  Saturation=sat  CoreLoss=Rm_phi0_1  BreakLoop=off  DiscreteSolver=Trapezoidal iterative  DataType=off  InitialFlux=-4.6560781327893e-06  TransfoNumber=1
      settings: SourceProductName=Simscape Electrical  SourceProductBaseCode=PS
  A : PMIOPort  Side=Left
  B : PMIOPort  Port=2  Side=Left
  C : PMIOPort  Port=3  Side=Left
  a : PMIOPort  Port=4  Side=Right
  b : PMIOPort  Port=5  Side=Right
  c : PMIOPort  Port=6  Side=Right
  out : Outport  InitialOutput=0
  wires:
  Measurements/1(Out1) -> out/1
  connections:
  Ground3/LConn1 -- CT Burden/RConn1
  Ground4/LConn1 -- CT Burden1/RConn1
  Ground5/LConn1 -- CT Burden2/RConn1
  T1/RConn2 -- Ground1/LConn1
  T2/RConn2 -- Ground6/LConn1
  T3/RConn2 -- Ground2/LConn1
  CT Burden/LConn1 -- Measurements/RConn1
  CT Burden1/LConn1 -- Measurements/RConn2
  CT Burden2/LConn1 -- Measurements/RConn3
  T1/RConn1 -- Measurements/LConn1
  Measurements/LConn2 -- T2/RConn1
  Measurements/LConn3 -- T3/RConn1
  T1/LConn1 -- A/RConn1
  T2/LConn1 -- B/RConn1
  T3/LConn1 -- C/RConn1
  T3/LConn2 -- c/RConn1
  T2/LConn2 -- b/RConn1
  T1/LConn2 -- a/RConn1

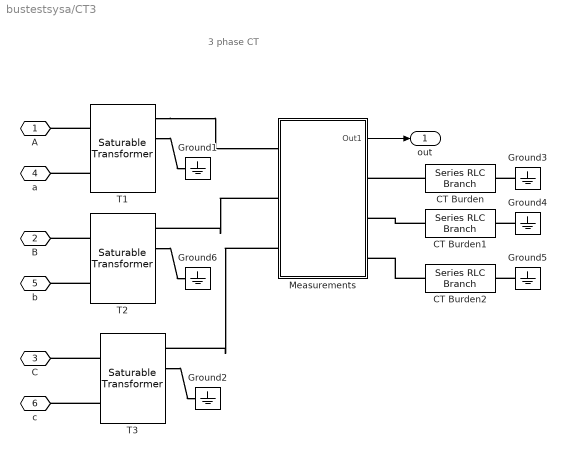
== system bustestsysa/CT3 ==
  note: 3 phase CT
  CT Burden : powerlib/Elements/Series RLC Branch  LConnTagsString=__new0  RConnTagsString=__new0  BranchType=RL  Resistance=3  Inductance=1e-3  SetiL0=off  InitialCurrent=0  Capacitance=1e-6  Setx0=off  InitialVoltage=0  Measurements=None
      settings: SourceProductName=Simscape Electrical
  CT Burden1 : powerlib/Elements/Series RLC Branch  LConnTagsString=__new0  RConnTagsString=__new0  BranchType=RL  Resistance=3  Inductance=1e-3  SetiL0=off  InitialCurrent=0  Capacitance=1e-6  Setx0=off  InitialVoltage=0  Measurements=None
      settings: SourceProductName=Simscape Electrical
  CT Burden2 : powerlib/Elements/Series RLC Branch  LConnTagsString=__new0  RConnTagsString=__new0  BranchType=RL  Resistance=3  Inductance=1e-3  SetiL0=off  InitialCurrent=0  Capacitance=1e-6  Setx0=off  InitialVoltage=0  Measurements=None
      settings: SourceProductName=Simscape Electrical
  Ground{1..6} (6 alike) : powerlib/Elements/Ground  LConnTagsString=a
      settings: SourceProductName=Simscape Electrical
  Measurements : Subsystem  mask(3 Phase Current Measurement){}
  T1 : powerlib/Elements/Saturable Transformer  ThreeWindings=off  Hysteresis=off  DataFile='hysteresis.mat'  Measurements=None  UNITS=pu  NominalPower=[pnom fnom]  Winding1=[u1 r1 x1]  Winding2=[u2 r2 x2]  Winding3=0  Saturation=sat  CoreLoss=Rm_phi0_1  BreakLoop=off  DiscreteSolver=Trapezoidal iterative  DataType=off  InitialFlux=0.000175463415264384  TransfoNumber=1
      settings: SourceProductName=Simscape Electrical  SourceProductBaseCode=PS
  T2 : powerlib/Elements/Saturable Transformer  ThreeWindings=off  Hysteresis=off  DataFile='hysteresis.mat'  Measurements=None  UNITS=pu  NominalPower=[pnom fnom]  Winding1=[u1 r1 x1]  Winding2=[u2 r2 x2]  Winding3=[u2 r2 x2]  Saturation=sat  CoreLoss=Rm_phi0_1  BreakLoop=off  DiscreteSolver=Trapezoidal iterative  DataType=off  InitialFlux=0.000528546466430355  TransfoNumber=1
      settings: SourceProductName=Simscape Electrical  SourceProductBaseCode=PS
  T3 : powerlib/Elements/Saturable Transformer  ThreeWindings=off  Hysteresis=off  DataFile='hysteresis.mat'  Measurements=None  UNITS=pu  NominalPower=[pnom fnom]  Winding1=[u1 r1 x1]  Winding2=[u2 r2 x2]  Winding3=[u2 r2 x2]  Saturation=sat  CoreLoss=Rm_phi0_1  BreakLoop=off  DiscreteSolver=Trapezoidal iterative  DataType=off  InitialFlux=-0.000704009881694765  TransfoNumber=1
      settings: SourceProductName=Simscape Electrical  SourceProductBaseCode=PS
  A : PMIOPort  Side=Left
  B : PMIOPort  Port=2  Side=Left
  C : PMIOPort  Port=3  Side=Left
  a : PMIOPort  Port=4  Side=Right
  b : PMIOPort  Port=5  Side=Right
  c : PMIOPort  Port=6  Side=Right
  out : Outport  InitialOutput=0
  wires:
  Measurements/1(Out1) -> out/1
  connections:
  Ground3/LConn1 -- CT Burden/RConn1
  Ground4/LConn1 -- CT Burden1/RConn1
  Ground5/LConn1 -- CT Burden2/RConn1
  T1/RConn2 -- Ground1/LConn1
  T2/RConn2 -- Ground6/LConn1
  T3/RConn2 -- Ground2/LConn1
  CT Burden/LConn1 -- Measurements/RConn1
  CT Burden1/LConn1 -- Measurements/RConn2
  CT Burden2/LConn1 -- Measurements/RConn3
  T1/RConn1 -- Measurements/LConn1
  Measurements/LConn2 -- T2/RConn1
  Measurements/LConn3 -- T3/RConn1
  T1/LConn1 -- A/RConn1
  T2/LConn1 -- B/RConn1
  T3/LConn1 -- C/RConn1
  T3/LConn2 -- c/RConn1
  T2/LConn2 -- b/RConn1
  T1/LConn2 -- a/RConn1

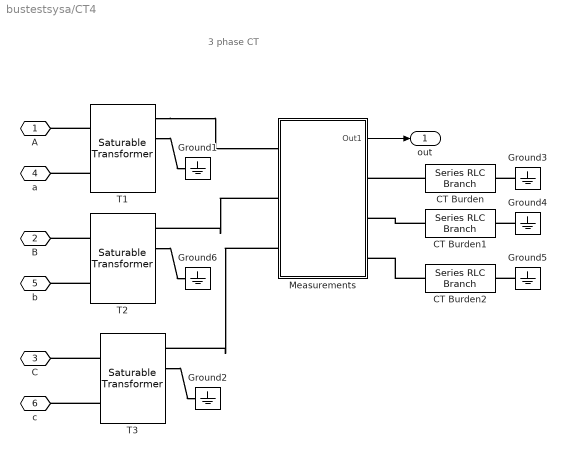
== system bustestsysa/CT4 ==
  note: 3 phase CT
  CT Burden : powerlib/Elements/Series RLC Branch  LConnTagsString=__new0  RConnTagsString=__new0  BranchType=RL  Resistance=3  Inductance=1e-3  SetiL0=off  InitialCurrent=0  Capacitance=1e-6  Setx0=off  InitialVoltage=0  Measurements=None
      settings: SourceProductName=Simscape Electrical
  CT Burden1 : powerlib/Elements/Series RLC Branch  LConnTagsString=__new0  RConnTagsString=__new0  BranchType=RL  Resistance=3  Inductance=1e-3  SetiL0=off  InitialCurrent=0  Capacitance=1e-6  Setx0=off  InitialVoltage=0  Measurements=None
      settings: SourceProductName=Simscape Electrical
  CT Burden2 : powerlib/Elements/Series RLC Branch  LConnTagsString=__new0  RConnTagsString=__new0  BranchType=RL  Resistance=3  Inductance=1e-3  SetiL0=off  InitialCurrent=0  Capacitance=1e-6  Setx0=off  InitialVoltage=0  Measurements=None
      settings: SourceProductName=Simscape Electrical
  Ground{1..6} (6 alike) : powerlib/Elements/Ground  LConnTagsString=a
      settings: SourceProductName=Simscape Electrical
  Measurements : Subsystem  mask(3 Phase Current Measurement){}
  T1 : powerlib/Elements/Saturable Transformer  ThreeWindings=off  Hysteresis=off  DataFile='hysteresis.mat'  Measurements=None  UNITS=pu  NominalPower=[pnom fnom]  Winding1=[u1 r1 x1]  Winding2=[u2 r2 x2]  Winding3=0  Saturation=sat  CoreLoss=Rm_phi0_1  BreakLoop=off  DiscreteSolver=Trapezoidal iterative  DataType=off  InitialFlux=-0.000150905892357555  TransfoNumber=1
      settings: SourceProductName=Simscape Electrical  SourceProductBaseCode=PS
  T2 : powerlib/Elements/Saturable Transformer  ThreeWindings=off  Hysteresis=off  DataFile='hysteresis.mat'  Measurements=None  UNITS=pu  NominalPower=[pnom fnom]  Winding1=[u1 r1 x1]  Winding2=[u2 r2 x2]  Winding3=[u2 r2 x2]  Saturation=sat  CoreLoss=Rm_phi0_1  BreakLoop=off  DiscreteSolver=Trapezoidal iterative  DataType=off  InitialFlux=-0.00012971098608721  TransfoNumber=1
      settings: SourceProductName=Simscape Electrical  SourceProductBaseCode=PS
  T3 : powerlib/Elements/Saturable Transformer  ThreeWindings=off  Hysteresis=off  DataFile='hysteresis.mat'  Measurements=None  UNITS=pu  NominalPower=[pnom fnom]  Winding1=[u1 r1 x1]  Winding2=[u2 r2 x2]  Winding3=[u2 r2 x2]  Saturation=sat  CoreLoss=Rm_phi0_1  BreakLoop=off  DiscreteSolver=Trapezoidal iterative  DataType=off  InitialFlux=0.000280616878444769  TransfoNumber=1
      settings: SourceProductName=Simscape Electrical  SourceProductBaseCode=PS
  A : PMIOPort  Side=Left
  B : PMIOPort  Port=2  Side=Left
  C : PMIOPort  Port=3  Side=Left
  a : PMIOPort  Port=4  Side=Right
  b : PMIOPort  Port=5  Side=Right
  c : PMIOPort  Port=6  Side=Right
  out : Outport  InitialOutput=0
  wires:
  Measurements/1(Out1) -> out/1
  connections:
  Ground3/LConn1 -- CT Burden/RConn1
  Ground4/LConn1 -- CT Burden1/RConn1
  Ground5/LConn1 -- CT Burden2/RConn1
  T1/RConn2 -- Ground1/LConn1
  T2/RConn2 -- Ground6/LConn1
  T3/RConn2 -- Ground2/LConn1
  CT Burden/LConn1 -- Measurements/RConn1
  CT Burden1/LConn1 -- Measurements/RConn2
  CT Burden2/LConn1 -- Measurements/RConn3
  T1/RConn1 -- Measurements/LConn1
  Measurements/LConn2 -- T2/RConn1
  Measurements/LConn3 -- T3/RConn1
  T1/LConn1 -- A/RConn1
  T2/LConn1 -- B/RConn1
  T3/LConn1 -- C/RConn1
  T3/LConn2 -- c/RConn1
  T2/LConn2 -- b/RConn1
  T1/LConn2 -- a/RConn1

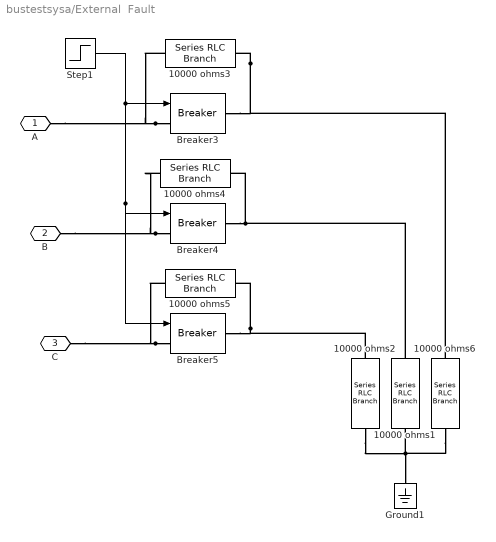
== system bustestsysa/External  Fault ==
  10000 ohms1 : powerlib/Elements/Series RLC Branch  LConnTagsString=__new0  RConnTagsString=__new0  BranchType=R  Resistance=1  Inductance=1e-3  SetiL0=off  InitialCurrent=0  Capacitance=1e-6  Setx0=off  InitialVoltage=0  Measurements=None
      settings: SourceProductName=Simscape Electrical
  10000 ohms2 : powerlib/Elements/Series RLC Branch  LConnTagsString=__new0  RConnTagsString=__new0  BranchType=R  Resistance=1  Inductance=1e-3  SetiL0=off  InitialCurrent=0  Capacitance=1e-6  Setx0=off  InitialVoltage=0  Measurements=None
      settings: SourceProductName=Simscape Electrical
  10000 ohms3 : powerlib/Elements/Series RLC Branch  LConnTagsString=__new0  RConnTagsString=__new0  BranchType=R  Resistance=10000  Inductance=1e-3  SetiL0=off  InitialCurrent=0  Capacitance=1e-6  Setx0=off  InitialVoltage=0  Measurements=None
      settings: SourceProductName=Simscape Electrical
  10000 ohms4 : powerlib/Elements/Series RLC Branch  LConnTagsString=__new0  RConnTagsString=__new0  BranchType=R  Resistance=10000  Inductance=1e-3  SetiL0=off  InitialCurrent=0  Capacitance=1e-6  Setx0=off  InitialVoltage=0  Measurements=None
      settings: SourceProductName=Simscape Electrical
  10000 ohms5 : powerlib/Elements/Series RLC Branch  LConnTagsString=__new0  RConnTagsString=__new0  BranchType=R  Resistance=10000  Inductance=1e-3  SetiL0=off  InitialCurrent=0  Capacitance=1e-6  Setx0=off  InitialVoltage=0  Measurements=None
      settings: SourceProductName=Simscape Electrical
  10000 ohms6 : powerlib/Elements/Series RLC Branch  LConnTagsString=__new0  RConnTagsString=__new0  BranchType=R  Resistance=1  Inductance=1e-3  SetiL0=off  InitialCurrent=0  Capacitance=1e-6  Setx0=off  InitialVoltage=0  Measurements=None
      settings: SourceProductName=Simscape Electrical
  Breaker3 : powerlib/Elements/Breaker  InitialState=0  SwitchingTimes="[ 1/60  5/60 ]"  External=on  BreakerResistance=0.01  SnubberResistance=1e6  SnubberCapacitance=inf  Measurements=None  MoreParameters=off  NoBreakLoop=off
      settings: SourceProductName=Simscape Electrical
  Breaker4 : powerlib/Elements/Breaker  InitialState=0  SwitchingTimes="[ 1/60  5/60 ]"  External=on  BreakerResistance=0.01  SnubberResistance=1e6  SnubberCapacitance=inf  Measurements=None  MoreParameters=off  NoBreakLoop=off
      settings: SourceProductName=Simscape Electrical
  Breaker5 : powerlib/Elements/Breaker  InitialState=0  SwitchingTimes="[ 1/60  5/60 ]"  External=on  BreakerResistance=0.01  SnubberResistance=1e6  SnubberCapacitance=inf  Measurements=None  MoreParameters=off  NoBreakLoop=off
      settings: SourceProductName=Simscape Electrical
  Ground1 : powerlib/Elements/Ground  LConnTagsString=a
      settings: SourceProductName=Simscape Electrical
  Step1 : Step  Time=Tfault  SampleTime=0
  A : PMIOPort  Side=Left
  B : PMIOPort  Port=2  Side=Left
  C : PMIOPort  Port=3  Side=Left
  wires:
  Step1/1 -> Breaker3/1, Breaker4/1, Breaker5/1
  connections:
  Breaker3/LConn1 -- 10000 ohms3/LConn1 -- A/RConn1
  10000 ohms6/LConn1 -- 10000 ohms3/RConn1 -- Breaker3/RConn1
  Breaker4/LConn1 -- 10000 ohms4/LConn1 -- B/RConn1
  10000 ohms1/LConn1 -- 10000 ohms4/RConn1 -- Breaker4/RConn1
  Breaker5/LConn1 -- 10000 ohms5/LConn1 -- C/RConn1
  10000 ohms2/LConn1 -- 10000 ohms5/RConn1 -- Breaker5/RConn1
  10000 ohms2/RConn1 -- 10000 ohms1/RConn1 -- 10000 ohms6/RConn1 -- Ground1/LConn1

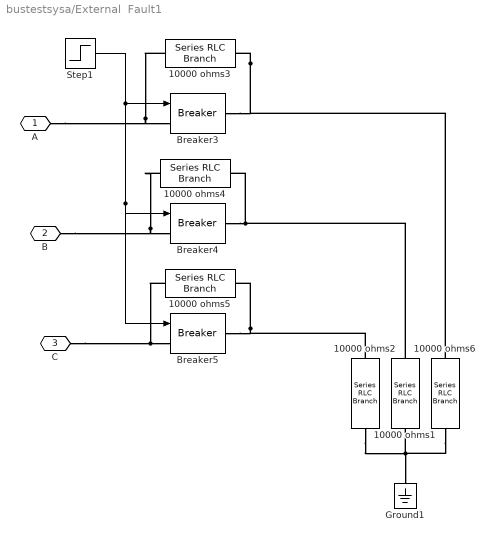
== system bustestsysa/External  Fault1 ==
  10000 ohms1 : powerlib/Elements/Series RLC Branch  LConnTagsString=__new0  RConnTagsString=__new0  BranchType=R  Resistance=1  Inductance=1e-3  SetiL0=off  InitialCurrent=0  Capacitance=1e-6  Setx0=off  InitialVoltage=0  Measurements=None
      settings: SourceProductName=Simscape Electrical
  10000 ohms2 : powerlib/Elements/Series RLC Branch  LConnTagsString=__new0  RConnTagsString=__new0  BranchType=R  Resistance=1  Inductance=1e-3  SetiL0=off  InitialCurrent=0  Capacitance=1e-6  Setx0=off  InitialVoltage=0  Measurements=None
      settings: SourceProductName=Simscape Electrical
  10000 ohms3 : powerlib/Elements/Series RLC Branch  LConnTagsString=__new0  RConnTagsString=__new0  BranchType=R  Resistance=10000  Inductance=1e-3  SetiL0=off  InitialCurrent=0  Capacitance=1e-6  Setx0=off  InitialVoltage=0  Measurements=None
      settings: SourceProductName=Simscape Electrical
  10000 ohms4 : powerlib/Elements/Series RLC Branch  LConnTagsString=__new0  RConnTagsString=__new0  BranchType=R  Resistance=10000  Inductance=1e-3  SetiL0=off  InitialCurrent=0  Capacitance=1e-6  Setx0=off  InitialVoltage=0  Measurements=None
      settings: SourceProductName=Simscape Electrical
  10000 ohms5 : powerlib/Elements/Series RLC Branch  LConnTagsString=__new0  RConnTagsString=__new0  BranchType=R  Resistance=10000  Inductance=1e-3  SetiL0=off  InitialCurrent=0  Capacitance=1e-6  Setx0=off  InitialVoltage=0  Measurements=None
      settings: SourceProductName=Simscape Electrical
  10000 ohms6 : powerlib/Elements/Series RLC Branch  LConnTagsString=__new0  RConnTagsString=__new0  BranchType=R  Resistance=1  Inductance=1e-3  SetiL0=off  InitialCurrent=0  Capacitance=1e-6  Setx0=off  InitialVoltage=0  Measurements=None
      settings: SourceProductName=Simscape Electrical
  Breaker3 : powerlib/Elements/Breaker  InitialState=0  SwitchingTimes="[ 1/60  5/60 ]"  External=on  BreakerResistance=0.01  SnubberResistance=1e6  SnubberCapacitance=inf  Measurements=None  MoreParameters=off  NoBreakLoop=off
      settings: SourceProductName=Simscape Electrical
  Breaker4 : powerlib/Elements/Breaker  InitialState=0  SwitchingTimes="[ 1/60  5/60 ]"  External=on  BreakerResistance=0.01  SnubberResistance=1e6  SnubberCapacitance=inf  Measurements=None  MoreParameters=off  NoBreakLoop=off
      settings: SourceProductName=Simscape Electrical
  Breaker5 : powerlib/Elements/Breaker  InitialState=0  SwitchingTimes="[ 1/60  5/60 ]"  External=on  BreakerResistance=0.01  SnubberResistance=1e6  SnubberCapacitance=inf  Measurements=None  MoreParameters=off  NoBreakLoop=off
      settings: SourceProductName=Simscape Electrical
  Ground1 : powerlib/Elements/Ground  LConnTagsString=a
      settings: SourceProductName=Simscape Electrical
  Step1 : Step  Time=Tfault  SampleTime=0
  A : PMIOPort  Side=Left
  B : PMIOPort  Port=2  Side=Left
  C : PMIOPort  Port=3  Side=Left
  wires:
  Step1/1 -> Breaker3/1, Breaker4/1, Breaker5/1
  connections:
  A/RConn1 -- Breaker3/LConn1 -- 10000 ohms3/LConn1
  Breaker3/RConn1 -- 10000 ohms6/LConn1 -- 10000 ohms3/RConn1
  B/RConn1 -- Breaker4/LConn1 -- 10000 ohms4/LConn1
  Breaker4/RConn1 -- 10000 ohms1/LConn1 -- 10000 ohms4/RConn1
  C/RConn1 -- Breaker5/LConn1 -- 10000 ohms5/LConn1
  Breaker5/RConn1 -- 10000 ohms2/LConn1 -- 10000 ohms5/RConn1
  10000 ohms2/RConn1 -- 10000 ohms1/RConn1 -- 10000 ohms6/RConn1 -- Ground1/LConn1

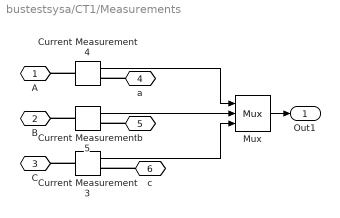
== system bustestsysa/CT1/Measurements ==
  Current Measurement3 : powerlib/Measurements/Current Measurement  PhasorSimulation=off  OutputType=Complex  PSBequivalent=0
      settings: SourceProductName=Simscape Electrical
  Current Measurement4 : powerlib/Measurements/Current Measurement  PhasorSimulation=off  OutputType=Complex  PSBequivalent=0
      settings: SourceProductName=Simscape Electrical
  Current Measurement5 : powerlib/Measurements/Current Measurement  PhasorSimulation=off  OutputType=Complex  PSBequivalent=0
      settings: SourceProductName=Simscape Electrical
  Mux : Mux  Inputs=3
  A : PMIOPort  Side=Left
  B : PMIOPort  Port=2  Side=Left
  C : PMIOPort  Port=3  Side=Left
  a : PMIOPort  Port=4  Side=Right
  b : PMIOPort  Port=5  Side=Right
  c : PMIOPort  Port=6  Side=Right
  Out1 : Outport  InitialOutput=0
  wires:
  Current Measurement4/1 -> Mux/1
  Current Measurement5/1 -> Mux/2
  Current Measurement3/1 -> Mux/3
  Mux/1 -> Out1/1
  connections:
  c/RConn1 -- Current Measurement3/RConn1
  b/RConn1 -- Current Measurement5/RConn1
  a/RConn1 -- Current Measurement4/RConn1
  Current Measurement4/LConn1 -- A/RConn1
  Current Measurement5/LConn1 -- B/RConn1
  Current Measurement3/LConn1 -- C/RConn1

== system bustestsysa/CT2/Measurements ==
  Current Measurement3 : powerlib/Measurements/Current Measurement  PhasorSimulation=off  OutputType=Complex  PSBequivalent=0
      settings: SourceProductName=Simscape Electrical
  Current Measurement4 : powerlib/Measurements/Current Measurement  PhasorSimulation=off  OutputType=Complex  PSBequivalent=0
      settings: SourceProductName=Simscape Electrical
  Current Measurement5 : powerlib/Measurements/Current Measurement  PhasorSimulation=off  OutputType=Complex  PSBequivalent=0
      settings: SourceProductName=Simscape Electrical
  Mux : Mux  Inputs=3
  A : PMIOPort  Side=Left
  B : PMIOPort  Port=2  Side=Left
  C : PMIOPort  Port=3  Side=Left
  a : PMIOPort  Port=4  Side=Right
  b : PMIOPort  Port=5  Side=Right
  c : PMIOPort  Port=6  Side=Right
  Out1 : Outport  InitialOutput=0
  wires:
  Current Measurement4/1 -> Mux/1
  Current Measurement5/1 -> Mux/2
  Current Measurement3/1 -> Mux/3
  Mux/1 -> Out1/1
  connections:
  c/RConn1 -- Current Measurement3/RConn1
  b/RConn1 -- Current Measurement5/RConn1
  a/RConn1 -- Current Measurement4/RConn1
  Current Measurement4/LConn1 -- A/RConn1
  Current Measurement5/LConn1 -- B/RConn1
  Current Measurement3/LConn1 -- C/RConn1

== system bustestsysa/CT3/Measurements ==
  Current Measurement3 : powerlib/Measurements/Current Measurement  PhasorSimulation=off  OutputType=Complex  PSBequivalent=0
      settings: SourceProductName=Simscape Electrical
  Current Measurement4 : powerlib/Measurements/Current Measurement  PhasorSimulation=off  OutputType=Complex  PSBequivalent=0
      settings: SourceProductName=Simscape Electrical
  Current Measurement5 : powerlib/Measurements/Current Measurement  PhasorSimulation=off  OutputType=Complex  PSBequivalent=0
      settings: SourceProductName=Simscape Electrical
  Mux : Mux  Inputs=3
  A : PMIOPort  Side=Left
  B : PMIOPort  Port=2  Side=Left
  C : PMIOPort  Port=3  Side=Left
  a : PMIOPort  Port=4  Side=Right
  b : PMIOPort  Port=5  Side=Right
  c : PMIOPort  Port=6  Side=Right
  Out1 : Outport  InitialOutput=0
  wires:
  Current Measurement4/1 -> Mux/1
  Current Measurement5/1 -> Mux/2
  Current Measurement3/1 -> Mux/3
  Mux/1 -> Out1/1
  connections:
  c/RConn1 -- Current Measurement3/RConn1
  b/RConn1 -- Current Measurement5/RConn1
  a/RConn1 -- Current Measurement4/RConn1
  Current Measurement4/LConn1 -- A/RConn1
  Current Measurement5/LConn1 -- B/RConn1
  Current Measurement3/LConn1 -- C/RConn1

== system bustestsysa/CT4/Measurements ==
  Current Measurement3 : powerlib/Measurements/Current Measurement  PhasorSimulation=off  OutputType=Complex  PSBequivalent=0
      settings: SourceProductName=Simscape Electrical
  Current Measurement4 : powerlib/Measurements/Current Measurement  PhasorSimulation=off  OutputType=Complex  PSBequivalent=0
      settings: SourceProductName=Simscape Electrical
  Current Measurement5 : powerlib/Measurements/Current Measurement  PhasorSimulation=off  OutputType=Complex  PSBequivalent=0
      settings: SourceProductName=Simscape Electrical
  Mux : Mux  Inputs=3
  A : PMIOPort  Side=Left
  B : PMIOPort  Port=2  Side=Left
  C : PMIOPort  Port=3  Side=Left
  a : PMIOPort  Port=4  Side=Right
  b : PMIOPort  Port=5  Side=Right
  c : PMIOPort  Port=6  Side=Right
  Out1 : Outport  InitialOutput=0
  wires:
  Current Measurement4/1 -> Mux/1
  Current Measurement5/1 -> Mux/2
  Current Measurement3/1 -> Mux/3
  Mux/1 -> Out1/1
  connections:
  c/RConn1 -- Current Measurement3/RConn1
  b/RConn1 -- Current Measurement5/RConn1
  a/RConn1 -- Current Measurement4/RConn1
  Current Measurement4/LConn1 -- A/RConn1
  Current Measurement5/LConn1 -- B/RConn1
  Current Measurement3/LConn1 -- C/RConn1
